simulink model "MJAUV_Maneuverability_model_V2"  (R2022b)
settings: Solver=ode4  StartTime=0.0  StopTime=50  FixedStep=0.0001  RelTol=1e-3  EnableMultiTasking=on
libraries: sharedutil x64, matrix_library x35
(part 4 of 5)

== system MJAUV_Maneuverability_model_V2/MJ-AUV Model & PropulsionSystem/Dynamics and Kinematics/Subsystem7/Rigid-body Coriolis and centripetal matrix1/Skew Symmetrical Operator  ==
  v : Inport
  Constant : Constant  Value=0
  Create 3x3 Matrix : sharedutil/Create 3x3 Matrix  aMode=aMode
  Demux : Demux  Outputs=3
      settings: DisplayOption=none
  Gain : Gain  Gain=-1  SaturateOnIntegerOverflow=on  OutDataTypeStr=Inherit: Same as input  ParamDataTypeStr=Inherit: Same as input
  Gain1 : Gain  Gain=-1  SaturateOnIntegerOverflow=on  OutDataTypeStr=Inherit: Same as input  ParamDataTypeStr=Inherit: Same as input
  Gain2 : Gain  Gain=-1  SaturateOnIntegerOverflow=on  OutDataTypeStr=Inherit: Same as input  ParamDataTypeStr=Inherit: Same as input
  S(V) : Outport  VectorParamsAs1DForOutWhenUnconnected=off
  wires:
  v/1 -> Demux/1
  Create 3x3 Matrix/1 -> S(V)/1
  Gain2/1 -> Create 3x3 Matrix/2  "-v(3)"
  Gain1/1 -> Create 3x3 Matrix/7  "-v(2)"
  Gain/1 -> Create 3x3 Matrix/6  "-v(1)"
  Demux/3 -> Create 3x3 Matrix/4, Gain2/1  "v(3)"
  Demux/2 -> Create 3x3 Matrix/3, Gain1/1  "v(2)"
  Demux/1 -> Create 3x3 Matrix/8, Gain/1  "v(1)"
  Constant/1 -> Create 3x3 Matrix/5, Create 3x3 Matrix/9, Create 3x3 Matrix/1

== system MJAUV_Maneuverability_model_V2/MJ-AUV Model & PropulsionSystem/Dynamics and Kinematics/Subsystem7/Rigid-body Coriolis and centripetal matrix1/Skew Symmetrical Operator ==
  v : Inport
  Constant : Constant  Value=0
  Create 3x3 Matrix : sharedutil/Create 3x3 Matrix  aMode=aMode
  Demux : Demux  Outputs=3
      settings: DisplayOption=none
  Gain : Gain  Gain=-1  SaturateOnIntegerOverflow=on  OutDataTypeStr=Inherit: Same as input  ParamDataTypeStr=Inherit: Same as input
  Gain1 : Gain  Gain=-1  SaturateOnIntegerOverflow=on  OutDataTypeStr=Inherit: Same as input  ParamDataTypeStr=Inherit: Same as input
  Gain2 : Gain  Gain=-1  SaturateOnIntegerOverflow=on  OutDataTypeStr=Inherit: Same as input  ParamDataTypeStr=Inherit: Same as input
  S(V) : Outport  VectorParamsAs1DForOutWhenUnconnected=off
  wires:
  v/1 -> Demux/1
  Create 3x3 Matrix/1 -> S(V)/1
  Gain2/1 -> Create 3x3 Matrix/2  "-v(3)"
  Gain1/1 -> Create 3x3 Matrix/7  "-v(2)"
  Gain/1 -> Create 3x3 Matrix/6  "-v(1)"
  Demux/3 -> Create 3x3 Matrix/4, Gain2/1  "v(3)"
  Demux/2 -> Create 3x3 Matrix/3, Gain1/1  "v(2)"
  Demux/1 -> Create 3x3 Matrix/8, Gain/1  "v(1)"
  Constant/1 -> Create 3x3 Matrix/5, Create 3x3 Matrix/9, Create 3x3 Matrix/1

== system MJAUV_Maneuverability_model_V2/MJ-AUV Model & PropulsionSystem/Dynamics and Kinematics/Subsystem7/Rigid-body Coriolis and centripetal matrix1/Skew Symmetrical Operator  ==
  v : Inport
  Constant : Constant  Value=0
  Create 3x3 Matrix : sharedutil/Create 3x3 Matrix  aMode=aMode
  Demux : Demux  Outputs=3
      settings: DisplayOption=none
  Gain : Gain  Gain=-1  SaturateOnIntegerOverflow=on  OutDataTypeStr=Inherit: Same as input  ParamDataTypeStr=Inherit: Same as input
  Gain1 : Gain  Gain=-1  SaturateOnIntegerOverflow=on  OutDataTypeStr=Inherit: Same as input  ParamDataTypeStr=Inherit: Same as input
  Gain2 : Gain  Gain=-1  SaturateOnIntegerOverflow=on  OutDataTypeStr=Inherit: Same as input  ParamDataTypeStr=Inherit: Same as input
  S(V) : Outport  VectorParamsAs1DForOutWhenUnconnected=off
  wires:
  Constant/1 -> Create 3x3 Matrix/1, Create 3x3 Matrix/9, Create 3x3 Matrix/5
  Demux/1 -> Gain/1, Create 3x3 Matrix/8  "v(1)"
  Demux/2 -> Gain1/1, Create 3x3 Matrix/3  "v(2)"
  Demux/3 -> Gain2/1, Create 3x3 Matrix/4  "v(3)"
  Gain/1 -> Create 3x3 Matrix/6  "-v(1)"
  Gain1/1 -> Create 3x3 Matrix/7  "-v(2)"
  Gain2/1 -> Create 3x3 Matrix/2  "-v(3)"
  Create 3x3 Matrix/1 -> S(V)/1
  v/1 -> Demux/1

== system MJAUV_Maneuverability_model_V2/MJ-AUV Model & PropulsionSystem/Dynamics and Kinematics/Subsystem7/Rigid-body Coriolis and centripetal matrix1/Skew Symmetrical Operator   ==
  v : Inport
  Constant : Constant  Value=0
  Create 3x3 Matrix : sharedutil/Create 3x3 Matrix  aMode=aMode
  Demux : Demux  Outputs=3
      settings: DisplayOption=none
  Gain : Gain  Gain=-1  SaturateOnIntegerOverflow=on  OutDataTypeStr=Inherit: Same as input  ParamDataTypeStr=Inherit: Same as input
  Gain1 : Gain  Gain=-1  SaturateOnIntegerOverflow=on  OutDataTypeStr=Inherit: Same as input  ParamDataTypeStr=Inherit: Same as input
  Gain2 : Gain  Gain=-1  SaturateOnIntegerOverflow=on  OutDataTypeStr=Inherit: Same as input  ParamDataTypeStr=Inherit: Same as input
  S(V) : Outport  VectorParamsAs1DForOutWhenUnconnected=off
  wires:
  v/1 -> Demux/1
  Create 3x3 Matrix/1 -> S(V)/1
  Gain2/1 -> Create 3x3 Matrix/2  "-v(3)"
  Gain1/1 -> Create 3x3 Matrix/7  "-v(2)"
  Gain/1 -> Create 3x3 Matrix/6  "-v(1)"
  Demux/3 -> Create 3x3 Matrix/4, Gain2/1  "v(3)"
  Demux/2 -> Create 3x3 Matrix/3, Gain1/1  "v(2)"
  Demux/1 -> Create 3x3 Matrix/8, Gain/1  "v(1)"
  Constant/1 -> Create 3x3 Matrix/5, Create 3x3 Matrix/9, Create 3x3 Matrix/1

== system MJAUV_Maneuverability_model_V2/MJ-AUV Model & PropulsionSystem/Dynamics and Kinematics/Subsystem7/Rigid-body Coriolis and centripetal matrix1/Subsystem ==
  rG_T : Inport
  Add : Sum
  Constant2 : Constant  Value=IT
  Gain5 : Gain  Gain=-mT
  Matrix Multiply4 : Product  Multiplication=Matrix(*)
  Skew Symmetrical Operator1 : Subsystem
  Ib_T : Outport
  wires:
  rG_T/1 -> Skew Symmetrical Operator1/1(v)  "rG_T"
  Constant2/1 -> Add/1
  Gain5/1 -> Add/2
  Matrix Multiply4/1 -> Gain5/1
  Skew Symmetrical Operator1/1(S(V)) -> Matrix Multiply4/1, Matrix Multiply4/2  "skewsymm(rG_T)"
  Add/1 -> Ib_T/1  "Ib_T"

== system MJAUV_Maneuverability_model_V2/MJ-AUV Model & PropulsionSystem/Dynamics and Kinematics/Subsystem7/Subsystem1/Quaternion normalisation ==
  eta_E : Inport
  Mux : Mux  Inputs=2
  Product : Product  Inputs=*/  SaturateOnIntegerOverflow=on  OutDataTypeStr=Inherit: Same as first input
  Reshape : Reshape  OutputDimensionality=Column vector (2-D)
  Selector : Selector  InputPortWidth=7  IndexOptions=Index vector (dialog)  Indices=[1 2 3]  OutputSizes=1
  Selector1 : Selector  InputPortWidth=7  IndexOptions=Index vector (dialog)  Indices=[4 5 6 7]  OutputSizes=1
  norm 1x4 vector : Subsystem
  eta_E (norm) : Outport  VectorParamsAs1DForOutWhenUnconnected=off
  wires:
  norm 1x4 vector/1(norm) -> Product/2
  Reshape/1 -> eta_E (norm)/1
  Mux/1 -> Reshape/1
  Product/1 -> Mux/2
  Selector/1 -> Mux/1
  Selector1/1 -> Product/1, norm 1x4 vector/1(Inport)
  eta_E/1 -> Selector/1, Selector1/1  "eta_E"

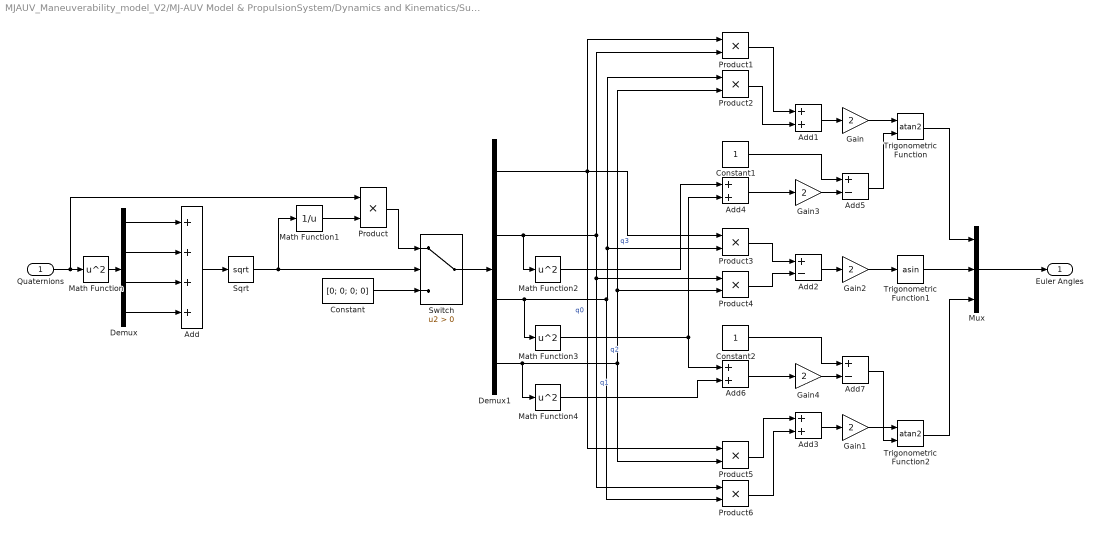
== system MJAUV_Maneuverability_model_V2/MJ-AUV Model & PropulsionSystem/Dynamics and Kinematics/Subsystem7/Subsystem1/Quaternions to Euler Angles ==
  Quaternions : Inport
  Add : Sum  Inputs=4
  Add{1,3..4,6} (4 alike) : Sum
  Add2 : Sum  Inputs=+-
  Add5 : Sum  Inputs=+-
  Add7 : Sum  Inputs=+-
  Constant : Constant  Value=[0; 0; 0; 0]
  Constant1 : Constant
  Constant2 : Constant
  Demux : Demux
  Demux1 : Demux
  Gain{,1..4} (5 alike) : Gain  Gain=2
  Math Function{,2..4} (4 alike) : Math  Operator=square  SignedPower=on
  Math Function1 : Math  Operator=reciprocal  SignedPower=on
  Mux : Mux  Inputs=3
  Product{,1..6} (7 alike) : Product
  Sqrt : Sqrt
  Switch : Switch  Criteria=u2 > Threshold  SaturateOnIntegerOverflow=off  InputSameDT=off
  Trigonometric Function : Trigonometry  Operator=atan2
  Trigonometric Function1 : Trigonometry  Operator=asin
  Trigonometric Function2 : Trigonometry  Operator=atan2
  Euler Angles : Outport  VectorParamsAs1DForOutWhenUnconnected=off
  wires:
  Quaternions/1 -> Product/1, Math Function/1
  Add/1 -> Sqrt/1
  Sqrt/1 -> Math Function1/1, Switch/2
  Constant/1 -> Switch/3
  Math Function1/1 -> Product/2
  Product/1 -> Switch/1
  Switch/1 -> Demux1/1
  Demux1/1 -> Product5/1, Product3/1, Product1/1  "q0"
  Demux1/2 -> Product6/1, Product4/1, Product1/2, Math Function2/1  "q1"
  Demux1/3 -> Product6/2, Product3/2, Product2/1, Math Function3/1  "q2"
  Demux1/4 -> Product5/2, Product4/2, Product2/2, Math Function4/1  "q3"
  Trigonometric Function1/1 -> Mux/2
  Mux/1 -> Euler Angles/1
  Trigonometric Function/1 -> Mux/1
  Trigonometric Function2/1 -> Mux/3
  Gain/1 -> Trigonometric Function/1
  Gain1/1 -> Trigonometric Function2/1
  Gain2/1 -> Trigonometric Function1/1
  Add1/1 -> Gain/1
  Add2/1 -> Gain2/1
  Add3/1 -> Gain1/1
  Product3/1 -> Add2/1
  Product4/1 -> Add2/2
  Product5/1 -> Add3/1
  Product6/1 -> Add3/2
  Product2/1 -> Add1/2
  Product1/1 -> Add1/1
  Add4/1 -> Gain3/1
  Gain3/1 -> Add5/2
  Constant1/1 -> Add5/1
  Add5/1 -> Trigonometric Function/2
  Add7/1 -> Trigonometric Function2/2
  Add6/1 -> Gain4/1
  Gain4/1 -> Add7/2
  Constant2/1 -> Add7/1
  Math Function2/1 -> Add4/1
  Math Function3/1 -> Add6/1, Add4/2
  Math Function4/1 -> Add6/2
  Demux/1 -> Add/1
  Demux/2 -> Add/2
  Demux/3 -> Add/3
  Demux/4 -> Add/4
  Math Function/1 -> Demux/1

== system MJAUV_Maneuverability_model_V2/MJ-AUV Model & PropulsionSystem/Dynamics and Kinematics/Subsystem7/Subsystem1/Subsystem ==
  "Euler Angles " : Inport
  Add : Sum
  Add1 : Sum  Inputs=-+
  Add2 : Sum
  Add3 : Sum  Inputs=+-
  Demux : Demux  Outputs=3
  Demux1 : Demux  Outputs=3
  Gain : Gain  Gain=0.5
  Mux : Mux
  Product{,1..7} (8 alike) : Product  Inputs=3
  Trigonometric Function : Trigonometry
  Trigonometric Function1 : Trigonometry  Operator=cos
  Quaternions : Outport  VectorParamsAs1DForOutWhenUnconnected=off
  wires:
  Add3/1 -> Mux/4
  Add2/1 -> Mux/3
  Add/1 -> Mux/1
  Add1/1 -> Mux/2
  Mux/1 -> Quaternions/1
  Product7/1 -> Add3/2
  Product6/1 -> Add3/1
  Product5/1 -> Add2/2
  Product4/1 -> Add2/1
  Product3/1 -> Add1/2
  Product2/1 -> Add1/1
  Product1/1 -> Add/2
  Product/1 -> Add/1
  Demux1/3 -> Product5/3, Product1/3, Product3/3, Product7/3  "cos(Y/2)"
  Demux1/1 -> Product5/1, Product2/1, Product1/1, Product6/1  "cos(R/2)"
  Demux1/2 -> Product6/2, Product1/2, Product3/2, Product4/2  "cos(P/2)"
  Trigonometric Function1/1 -> Demux1/1
  Demux/3 -> Product/3, Product2/3, Product4/3, Product6/3  "sin(Y/2)"
  Demux/2 -> Product/2, Product2/2, Product5/2, Product7/2  "sin(P/2)"
  Demux/1 -> Product/1, Product3/1, Product4/1, Product7/1  "sin(R/2)"
  Trigonometric Function/1 -> Demux/1
  Gain/1 -> Trigonometric Function/1, Trigonometric Function1/1
  "Euler Angles "/1 -> Gain/1

== system MJAUV_Maneuverability_model_V2/MJ-AUV Model & PropulsionSystem/Dynamics and Kinematics/Subsystem7/Subsystem1/Subsystem1 ==
  In2 : Inport
  Abs : Abs  SaturateOnIntegerOverflow=off
  Add : Sum  Inputs=-+
  Constant : Constant  Value=2*pi
  Switch : Switch  Criteria=u2 > Threshold  Threshold=pi  SaturateOnIntegerOverflow=off  InputSameDT=off
  Out1 : Outport
  wires:
  In2/1 -> Add/2, Switch/3, Abs/1
  Switch/1 -> Out1/1
  Add/1 -> Switch/1
  Abs/1 -> Switch/2
  Constant/1 -> Add/1

== system MJAUV_Maneuverability_model_V2/MJ-AUV Model & PropulsionSystem/Dynamics and Kinematics/Subsystem8/Added Mass Coriolis and centripetal matrix1/Skew Symmetrical Operator ==
  v : Inport
  Constant : Constant  Value=0
  Create 3x3 Matrix : sharedutil/Create 3x3 Matrix  aMode=aMode
  Demux : Demux  Outputs=3
      settings: DisplayOption=none
  Gain : Gain  Gain=-1  SaturateOnIntegerOverflow=on  OutDataTypeStr=Inherit: Same as input  ParamDataTypeStr=Inherit: Same as input
  Gain1 : Gain  Gain=-1  SaturateOnIntegerOverflow=on  OutDataTypeStr=Inherit: Same as input  ParamDataTypeStr=Inherit: Same as input
  Gain2 : Gain  Gain=-1  SaturateOnIntegerOverflow=on  OutDataTypeStr=Inherit: Same as input  ParamDataTypeStr=Inherit: Same as input
  S(V) : Outport  VectorParamsAs1DForOutWhenUnconnected=off
  wires:
  v/1 -> Demux/1
  Create 3x3 Matrix/1 -> S(V)/1
  Gain2/1 -> Create 3x3 Matrix/2  "-v(3)"
  Gain1/1 -> Create 3x3 Matrix/7  "-v(2)"
  Gain/1 -> Create 3x3 Matrix/6  "-v(1)"
  Demux/3 -> Create 3x3 Matrix/4, Gain2/1  "v(3)"
  Demux/2 -> Create 3x3 Matrix/3, Gain1/1  "v(2)"
  Demux/1 -> Create 3x3 Matrix/8, Gain/1  "v(1)"
  Constant/1 -> Create 3x3 Matrix/5, Create 3x3 Matrix/9, Create 3x3 Matrix/1

== system MJAUV_Maneuverability_model_V2/MJ-AUV Model & PropulsionSystem/Dynamics and Kinematics/Subsystem8/Added Mass Coriolis and centripetal matrix1/Skew Symmetrical Operator  ==
  v : Inport
  Constant : Constant  Value=0
  Create 3x3 Matrix : sharedutil/Create 3x3 Matrix  aMode=aMode
  Demux : Demux  Outputs=3
      settings: DisplayOption=none
  Gain : Gain  Gain=-1  SaturateOnIntegerOverflow=on  OutDataTypeStr=Inherit: Same as input  ParamDataTypeStr=Inherit: Same as input
  Gain1 : Gain  Gain=-1  SaturateOnIntegerOverflow=on  OutDataTypeStr=Inherit: Same as input  ParamDataTypeStr=Inherit: Same as input
  Gain2 : Gain  Gain=-1  SaturateOnIntegerOverflow=on  OutDataTypeStr=Inherit: Same as input  ParamDataTypeStr=Inherit: Same as input
  S(V) : Outport  VectorParamsAs1DForOutWhenUnconnected=off
  wires:
  Constant/1 -> Create 3x3 Matrix/1, Create 3x3 Matrix/9, Create 3x3 Matrix/5
  Demux/1 -> Gain/1, Create 3x3 Matrix/8  "v(1)"
  Demux/2 -> Gain1/1, Create 3x3 Matrix/3  "v(2)"
  Demux/3 -> Gain2/1, Create 3x3 Matrix/4  "v(3)"
  Gain/1 -> Create 3x3 Matrix/6  "-v(1)"
  Gain1/1 -> Create 3x3 Matrix/7  "-v(2)"
  Gain2/1 -> Create 3x3 Matrix/2  "-v(3)"
  Create 3x3 Matrix/1 -> S(V)/1
  v/1 -> Demux/1

== system MJAUV_Maneuverability_model_V2/MJ-AUV Model & PropulsionSystem/Dynamics and Kinematics/Subsystem8/Added Mass Coriolis and centripetal matrix1/Subsystem ==
  Create Diagonal Matrix1 : matrix_library/Create Diagonal Matrix
  K_pdot_F : Constant  Value=0
  M_qdot_F : Constant  Value=(pi*rho*R^2*LF^3)/12
  Mux : Mux  Inputs=6
  N_rdot_F : Constant  Value=(pi*rho*R^2*LF^3)/12
  Reshape1 : Reshape  OutputDimensionality=Column vector (2-D)  OutputDimensions=[6,6]
  X_udot_F : Constant  Value=0.1*mF
  Y_vdot_F : Constant  Value=pi*rho*R*R*LF
  Z_wdot_F : Constant  Value=pi*rho*R^2*LF
  MA_F : Outport
  wires:
  Create Diagonal Matrix1/1 -> MA_F/1
  K_pdot_F/1 -> Mux/4
  N_rdot_F/1 -> Mux/6
  M_qdot_F/1 -> Mux/5
  X_udot_F/1 -> Mux/1
  Y_vdot_F/1 -> Mux/2
  Reshape1/1 -> Create Diagonal Matrix1/1
  Mux/1 -> Reshape1/1
  Z_wdot_F/1 -> Mux/3

== system MJAUV_Maneuverability_model_V2/MJ-AUV Model & PropulsionSystem/Dynamics and Kinematics/Subsystem8/Restoring forces1/E1(e) ==
  e : Inport
  Gain : Gain  Gain=2  SaturateOnIntegerOverflow=on  OutDataTypeStr=Inherit: Same as input  ParamDataTypeStr=Inherit: Same as input
  "Gain " : Gain  Gain=2  SaturateOnIntegerOverflow=on  OutDataTypeStr=Inherit: Same as input  ParamDataTypeStr=Inherit: Same as input
  I (3x3) : Constant  Value=eye(3)
  Matrix Multiply : Product  Multiplication=Matrix(*)
  Product : Product  SaturateOnIntegerOverflow=on  OutDataTypeStr=Inherit: Same as first input
  Selector : Selector  InputPortWidth=4  IndexOptions=Index vector (dialog)  Indices=[1]  OutputSizes=1
  Selector1 : Selector  InputPortWidth=4  IndexOptions=Index vector (dialog)  Indices=[2 3 4]  OutputSizes=1
  Skew Symmetrical Operator : Subsystem
  Sum : Sum  Inputs=+++  SaturateOnIntegerOverflow=on
  E1 : Outport  VectorParamsAs1DForOutWhenUnconnected=off
  wires:
  Sum/1 -> E1/1
  Gain/1 -> Sum/3
  Product/1 -> Sum/2
  I (3x3)/1 -> Sum/1
  "Gain "/1 -> Product/1
  Matrix Multiply/1 -> Gain/1
  Skew Symmetrical Operator/1(S(V)) -> Product/2, Matrix Multiply/2, Matrix Multiply/1
  Selector1/1 -> Skew Symmetrical Operator/1(v)  "eps"
  Selector/1 -> "Gain "/1  "eta"
  e/1 -> Selector1/1, Selector/1

== system MJAUV_Maneuverability_model_V2/MJ-AUV Model & PropulsionSystem/Dynamics and Kinematics/Subsystem8/Rigid-body Coriolis and centripetal matrix1/Ib_F ==
  rG_F : Inport
  Add : Sum
  Constant2 : Constant  Value=IF
  Gain5 : Gain  Gain=-mF
  Matrix Multiply4 : Product  Multiplication=Matrix(*)
  Skew Symmetrical Operator1 : Subsystem
  Ib_F : Outport
  wires:
  rG_F/1 -> Skew Symmetrical Operator1/1(v)  "rG_F"
  Constant2/1 -> Add/1
  Gain5/1 -> Add/2
  Matrix Multiply4/1 -> Gain5/1
  Skew Symmetrical Operator1/1(S(V)) -> Matrix Multiply4/1, Matrix Multiply4/2  "skewsymm(rG_F)"
  Add/1 -> Ib_F/1  "Ib_F"

== system MJAUV_Maneuverability_model_V2/MJ-AUV Model & PropulsionSystem/Dynamics and Kinematics/Subsystem8/Rigid-body Coriolis and centripetal matrix1/Skew Symmetrical Operator  ==
  v : Inport
  Constant : Constant  Value=0
  Create 3x3 Matrix : sharedutil/Create 3x3 Matrix  aMode=aMode
  Demux : Demux  Outputs=3
      settings: DisplayOption=none
  Gain : Gain  Gain=-1  SaturateOnIntegerOverflow=on  OutDataTypeStr=Inherit: Same as input  ParamDataTypeStr=Inherit: Same as input
  Gain1 : Gain  Gain=-1  SaturateOnIntegerOverflow=on  OutDataTypeStr=Inherit: Same as input  ParamDataTypeStr=Inherit: Same as input
  Gain2 : Gain  Gain=-1  SaturateOnIntegerOverflow=on  OutDataTypeStr=Inherit: Same as input  ParamDataTypeStr=Inherit: Same as input
  S(V) : Outport  VectorParamsAs1DForOutWhenUnconnected=off
  wires:
  Constant/1 -> Create 3x3 Matrix/1, Create 3x3 Matrix/9, Create 3x3 Matrix/5
  Demux/1 -> Gain/1, Create 3x3 Matrix/8  "v(1)"
  Demux/2 -> Gain1/1, Create 3x3 Matrix/3  "v(2)"
  Demux/3 -> Gain2/1, Create 3x3 Matrix/4  "v(3)"
  Gain/1 -> Create 3x3 Matrix/6  "-v(1)"
  Gain1/1 -> Create 3x3 Matrix/7  "-v(2)"
  Gain2/1 -> Create 3x3 Matrix/2  "-v(3)"
  Create 3x3 Matrix/1 -> S(V)/1
  v/1 -> Demux/1

== system MJAUV_Maneuverability_model_V2/MJ-AUV Model & PropulsionSystem/Dynamics and Kinematics/Subsystem8/Rigid-body Coriolis and centripetal matrix1/Skew Symmetrical Operator ==
  v : Inport
  Constant : Constant  Value=0
  Create 3x3 Matrix : sharedutil/Create 3x3 Matrix  aMode=aMode
  Demux : Demux  Outputs=3
      settings: DisplayOption=none
  Gain : Gain  Gain=-1  SaturateOnIntegerOverflow=on  OutDataTypeStr=Inherit: Same as input  ParamDataTypeStr=Inherit: Same as input
  Gain1 : Gain  Gain=-1  SaturateOnIntegerOverflow=on  OutDataTypeStr=Inherit: Same as input  ParamDataTypeStr=Inherit: Same as input
  Gain2 : Gain  Gain=-1  SaturateOnIntegerOverflow=on  OutDataTypeStr=Inherit: Same as input  ParamDataTypeStr=Inherit: Same as input
  S(V) : Outport  VectorParamsAs1DForOutWhenUnconnected=off
  wires:
  Constant/1 -> Create 3x3 Matrix/1, Create 3x3 Matrix/9, Create 3x3 Matrix/5
  Demux/1 -> Gain/1, Create 3x3 Matrix/8  "v(1)"
  Demux/2 -> Gain1/1, Create 3x3 Matrix/3  "v(2)"
  Demux/3 -> Gain2/1, Create 3x3 Matrix/4  "v(3)"
  Gain/1 -> Create 3x3 Matrix/6  "-v(1)"
  Gain1/1 -> Create 3x3 Matrix/7  "-v(2)"
  Gain2/1 -> Create 3x3 Matrix/2  "-v(3)"
  Create 3x3 Matrix/1 -> S(V)/1
  v/1 -> Demux/1

== system MJAUV_Maneuverability_model_V2/MJ-AUV Model & PropulsionSystem/Dynamics and Kinematics/Subsystem8/Rigid-body Coriolis and centripetal matrix1/Skew Symmetrical Operator  ==
  v : Inport
  Constant : Constant  Value=0
  Create 3x3 Matrix : sharedutil/Create 3x3 Matrix  aMode=aMode
  Demux : Demux  Outputs=3
      settings: DisplayOption=none
  Gain : Gain  Gain=-1  SaturateOnIntegerOverflow=on  OutDataTypeStr=Inherit: Same as input  ParamDataTypeStr=Inherit: Same as input
  Gain1 : Gain  Gain=-1  SaturateOnIntegerOverflow=on  OutDataTypeStr=Inherit: Same as input  ParamDataTypeStr=Inherit: Same as input
  Gain2 : Gain  Gain=-1  SaturateOnIntegerOverflow=on  OutDataTypeStr=Inherit: Same as input  ParamDataTypeStr=Inherit: Same as input
  S(V) : Outport  VectorParamsAs1DForOutWhenUnconnected=off
  wires:
  v/1 -> Demux/1
  Create 3x3 Matrix/1 -> S(V)/1
  Gain2/1 -> Create 3x3 Matrix/2  "-v(3)"
  Gain1/1 -> Create 3x3 Matrix/7  "-v(2)"
  Gain/1 -> Create 3x3 Matrix/6  "-v(1)"
  Demux/3 -> Create 3x3 Matrix/4, Gain2/1  "v(3)"
  Demux/2 -> Create 3x3 Matrix/3, Gain1/1  "v(2)"
  Demux/1 -> Create 3x3 Matrix/8, Gain/1  "v(1)"
  Constant/1 -> Create 3x3 Matrix/5, Create 3x3 Matrix/9, Create 3x3 Matrix/1

== system MJAUV_Maneuverability_model_V2/MJ-AUV Model & PropulsionSystem/Dynamics and Kinematics/Subsystem8/Rigid-body Coriolis and centripetal matrix1/Skew Symmetrical Operator   ==
  v : Inport
  Constant : Constant  Value=0
  Create 3x3 Matrix : sharedutil/Create 3x3 Matrix  aMode=aMode
  Demux : Demux  Outputs=3
      settings: DisplayOption=none
  Gain : Gain  Gain=-1  SaturateOnIntegerOverflow=on  OutDataTypeStr=Inherit: Same as input  ParamDataTypeStr=Inherit: Same as input
  Gain1 : Gain  Gain=-1  SaturateOnIntegerOverflow=on  OutDataTypeStr=Inherit: Same as input  ParamDataTypeStr=Inherit: Same as input
  Gain2 : Gain  Gain=-1  SaturateOnIntegerOverflow=on  OutDataTypeStr=Inherit: Same as input  ParamDataTypeStr=Inherit: Same as input
  S(V) : Outport  VectorParamsAs1DForOutWhenUnconnected=off
  wires:
  Constant/1 -> Create 3x3 Matrix/1, Create 3x3 Matrix/9, Create 3x3 Matrix/5
  Demux/1 -> Gain/1, Create 3x3 Matrix/8  "v(1)"
  Demux/2 -> Gain1/1, Create 3x3 Matrix/3  "v(2)"
  Demux/3 -> Gain2/1, Create 3x3 Matrix/4  "v(3)"
  Gain/1 -> Create 3x3 Matrix/6  "-v(1)"
  Gain1/1 -> Create 3x3 Matrix/7  "-v(2)"
  Gain2/1 -> Create 3x3 Matrix/2  "-v(3)"
  Create 3x3 Matrix/1 -> S(V)/1
  v/1 -> Demux/1

== system MJAUV_Maneuverability_model_V2/MJ-AUV Model & PropulsionSystem/Dynamics and Kinematics/Subsystem8/Subsystem1/Quaternion normalisation ==
  eta_E : Inport
  Mux : Mux  Inputs=2
  Product : Product  Inputs=*/  SaturateOnIntegerOverflow=on  OutDataTypeStr=Inherit: Same as first input
  Reshape : Reshape  OutputDimensionality=Column vector (2-D)
  Selector : Selector  InputPortWidth=7  IndexOptions=Index vector (dialog)  Indices=[1 2 3]  OutputSizes=1
  Selector1 : Selector  InputPortWidth=7  IndexOptions=Index vector (dialog)  Indices=[4 5 6 7]  OutputSizes=1
  norm 1x4 vector : Subsystem
  eta_E (norm) : Outport  VectorParamsAs1DForOutWhenUnconnected=off
  wires:
  norm 1x4 vector/1(norm) -> Product/2
  Reshape/1 -> eta_E (norm)/1
  Mux/1 -> Reshape/1
  Product/1 -> Mux/2
  Selector/1 -> Mux/1
  Selector1/1 -> Product/1, norm 1x4 vector/1(Inport)
  eta_E/1 -> Selector/1, Selector1/1  "eta_E"

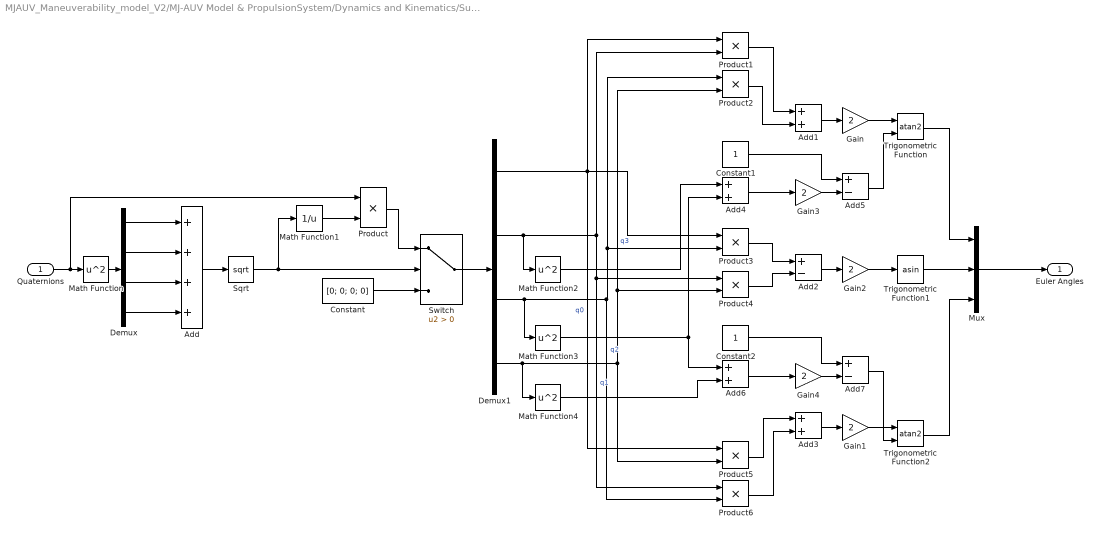
== system MJAUV_Maneuverability_model_V2/MJ-AUV Model & PropulsionSystem/Dynamics and Kinematics/Subsystem8/Subsystem1/Quaternions to Euler Angles ==
  Quaternions : Inport
  Add : Sum  Inputs=4
  Add{1,3..4,6} (4 alike) : Sum
  Add2 : Sum  Inputs=+-
  Add5 : Sum  Inputs=+-
  Add7 : Sum  Inputs=+-
  Constant : Constant  Value=[0; 0; 0; 0]
  Constant1 : Constant
  Constant2 : Constant
  Demux : Demux
  Demux1 : Demux
  Gain{,1..4} (5 alike) : Gain  Gain=2
  Math Function{,2..4} (4 alike) : Math  Operator=square  SignedPower=on
  Math Function1 : Math  Operator=reciprocal  SignedPower=on
  Mux : Mux  Inputs=3
  Product{,1..6} (7 alike) : Product
  Sqrt : Sqrt
  Switch : Switch  Criteria=u2 > Threshold  SaturateOnIntegerOverflow=off  InputSameDT=off
  Trigonometric Function : Trigonometry  Operator=atan2
  Trigonometric Function1 : Trigonometry  Operator=asin
  Trigonometric Function2 : Trigonometry  Operator=atan2
  Euler Angles : Outport  VectorParamsAs1DForOutWhenUnconnected=off
  wires:
  Quaternions/1 -> Product/1, Math Function/1
  Add/1 -> Sqrt/1
  Sqrt/1 -> Math Function1/1, Switch/2
  Constant/1 -> Switch/3
  Math Function1/1 -> Product/2
  Product/1 -> Switch/1
  Switch/1 -> Demux1/1
  Demux1/1 -> Product5/1, Product3/1, Product1/1  "q0"
  Demux1/2 -> Product6/1, Product4/1, Product1/2, Math Function2/1  "q1"
  Demux1/3 -> Product6/2, Product3/2, Product2/1, Math Function3/1  "q2"
  Demux1/4 -> Product5/2, Product4/2, Product2/2, Math Function4/1  "q3"
  Trigonometric Function1/1 -> Mux/2
  Mux/1 -> Euler Angles/1
  Trigonometric Function/1 -> Mux/1
  Trigonometric Function2/1 -> Mux/3
  Gain/1 -> Trigonometric Function/1
  Gain1/1 -> Trigonometric Function2/1
  Gain2/1 -> Trigonometric Function1/1
  Add1/1 -> Gain/1
  Add2/1 -> Gain2/1
  Add3/1 -> Gain1/1
  Product3/1 -> Add2/1
  Product4/1 -> Add2/2
  Product5/1 -> Add3/1
  Product6/1 -> Add3/2
  Product2/1 -> Add1/2
  Product1/1 -> Add1/1
  Add4/1 -> Gain3/1
  Gain3/1 -> Add5/2
  Constant1/1 -> Add5/1
  Add5/1 -> Trigonometric Function/2
  Add7/1 -> Trigonometric Function2/2
  Add6/1 -> Gain4/1
  Gain4/1 -> Add7/2
  Constant2/1 -> Add7/1
  Math Function2/1 -> Add4/1
  Math Function3/1 -> Add6/1, Add4/2
  Math Function4/1 -> Add6/2
  Demux/1 -> Add/1
  Demux/2 -> Add/2
  Demux/3 -> Add/3
  Demux/4 -> Add/4
  Math Function/1 -> Demux/1

== system MJAUV_Maneuverability_model_V2/MJ-AUV Model & PropulsionSystem/Dynamics and Kinematics/Subsystem8/Subsystem1/Subsystem ==
  "Euler Angles " : Inport
  Add : Sum
  Add1 : Sum  Inputs=-+
  Add2 : Sum
  Add3 : Sum  Inputs=+-
  Demux : Demux  Outputs=3
  Demux1 : Demux  Outputs=3
  Gain : Gain  Gain=0.5
  Mux : Mux
  Product{,1..7} (8 alike) : Product  Inputs=3
  Trigonometric Function : Trigonometry
  Trigonometric Function1 : Trigonometry  Operator=cos
  Quaternions : Outport  VectorParamsAs1DForOutWhenUnconnected=off
  wires:
  Add3/1 -> Mux/4
  Add2/1 -> Mux/3
  Add/1 -> Mux/1
  Add1/1 -> Mux/2
  Mux/1 -> Quaternions/1
  Product7/1 -> Add3/2
  Product6/1 -> Add3/1
  Product5/1 -> Add2/2
  Product4/1 -> Add2/1
  Product3/1 -> Add1/2
  Product2/1 -> Add1/1
  Product1/1 -> Add/2
  Product/1 -> Add/1
  Demux1/3 -> Product5/3, Product1/3, Product3/3, Product7/3  "cos(Y/2)"
  Demux1/1 -> Product5/1, Product2/1, Product1/1, Product6/1  "cos(R/2)"
  Demux1/2 -> Product6/2, Product1/2, Product3/2, Product4/2  "cos(P/2)"
  Trigonometric Function1/1 -> Demux1/1
  Demux/3 -> Product/3, Product2/3, Product4/3, Product6/3  "sin(Y/2)"
  Demux/2 -> Product/2, Product2/2, Product5/2, Product7/2  "sin(P/2)"
  Demux/1 -> Product/1, Product3/1, Product4/1, Product7/1  "sin(R/2)"
  Trigonometric Function/1 -> Demux/1
  Gain/1 -> Trigonometric Function/1, Trigonometric Function1/1
  "Euler Angles "/1 -> Gain/1

== system MJAUV_Maneuverability_model_V2/MJ-AUV Model & PropulsionSystem/Dynamics and Kinematics/Subsystem8/Subsystem1/Subsystem1 ==
  In2 : Inport
  Abs : Abs  SaturateOnIntegerOverflow=off
  Add : Sum  Inputs=-+
  Constant : Constant  Value=2*pi
  Switch : Switch  Criteria=u2 > Threshold  Threshold=pi  SaturateOnIntegerOverflow=off  InputSameDT=off
  Out1 : Outport
  wires:
  In2/1 -> Add/2, Switch/3, Abs/1
  Switch/1 -> Out1/1
  Add/1 -> Switch/1
  Abs/1 -> Switch/2
  Constant/1 -> Add/1

== system MJAUV_Maneuverability_model_V2/MJ-AUV Model & PropulsionSystem/Dynamics and Kinematics/Subsystem9/M_B/Subsystem ==
  Create Diagonal Matrix1 : matrix_library/Create Diagonal Matrix
  K_pdot_B : Constant  Value=0
  M_qdot_B : Constant  Value=(pi*rho*R^2*LB^3)/12
  Mux : Mux  Inputs=6
  N_rdot_B : Constant  Value=(pi*rho*R^2*LB^3)/12
  Reshape1 : Reshape  OutputDimensionality=Column vector (2-D)  OutputDimensions=[6,6]
  X_udot_B : Constant  Value=0.1*mB
  Y_vdot_B : Constant  Value=pi*rho*R*R*LB
  Z_wdot_B : Constant  Value=pi*rho*R^2*LB
  MA_B : Outport
  wires:
  Create Diagonal Matrix1/1 -> MA_B/1
  K_pdot_B/1 -> Mux/4
  N_rdot_B/1 -> Mux/6
  M_qdot_B/1 -> Mux/5
  X_udot_B/1 -> Mux/1
  Y_vdot_B/1 -> Mux/2
  Reshape1/1 -> Create Diagonal Matrix1/1
  Mux/1 -> Reshape1/1
  Z_wdot_B/1 -> Mux/3

== system MJAUV_Maneuverability_model_V2/MJ-AUV Model & PropulsionSystem/Dynamics and Kinematics/Subsystem9/M_B/Subsystem1 ==
  rG_B : Inport
  Add : Sum
  Constant2 : Constant  Value=IB
  Gain : Gain  Gain=-mB
  Gain1 : Gain  Gain=-1
  Gain2 : Gain  Gain=-mB
  Gain3 : Gain  Gain=mB
  Matrix Concatenation : Concatenate  Mode=Multidimensional array
  Matrix Concatenation1 : Concatenate  Mode=Multidimensional array
  Matrix Concatenation2 : Concatenate  Mode=Multidimensional array  ConcatenateDimension=2
  Matrix Multiply3 : Product  Multiplication=Matrix(*)
  Skew Symmetrical Operator1 : Subsystem
  eye(3,3) : Constant  Value=eye(3,3)
  MRB_B : Outport  VectorParamsAs1DForOutWhenUnconnected=off
  wires:
  Matrix Concatenation2/1 -> MRB_B/1
  Gain2/1 -> Add/2
  Skew Symmetrical Operator1/1(S(V)) -> Gain/1, Matrix Multiply3/2, Matrix Multiply3/1  "skewsymm(rG_B)"
  Gain3/1 -> Matrix Concatenation/1  "MRB_B(1,1)"
  eye(3,3)/1 -> Gain3/1  "eye(3,3)"
  Gain1/1 -> Matrix Concatenation1/1  "MRB_B(2,1)"
  Add/1 -> Matrix Concatenation1/2  "MRB_B(2,2)"
  Matrix Concatenation/1 -> Matrix Concatenation2/1
  Matrix Concatenation1/1 -> Matrix Concatenation2/2
  Gain/1 -> Matrix Concatenation/2, Gain1/1  "MRB_B(1,2)"
  Matrix Multiply3/1 -> Gain2/1
  Constant2/1 -> Add/1
  rG_B/1 -> Skew Symmetrical Operator1/1(v)

== system MJAUV_Maneuverability_model_V2/MJ-AUV Model & PropulsionSystem/Dynamics and Kinematics/Subsystem9/M_F/Subsystem ==
  Create Diagonal Matrix1 : matrix_library/Create Diagonal Matrix
  K_pdot_F : Constant  Value=0
  M_qdot_F : Constant  Value=(pi*rho*R^2*LF^3)/12
  Mux : Mux  Inputs=6
  N_rdot_F : Constant  Value=(pi*rho*R^2*LF^3)/12
  Reshape1 : Reshape  OutputDimensionality=Column vector (2-D)  OutputDimensions=[6,6]
  X_udot_F : Constant  Value=0.1*mF
  Y_vdot_F : Constant  Value=pi*rho*R*R*LF
  Z_wdot_F : Constant  Value=pi*rho*R^2*LF
  MA_F : Outport
  wires:
  Create Diagonal Matrix1/1 -> MA_F/1
  K_pdot_F/1 -> Mux/4
  N_rdot_F/1 -> Mux/6
  M_qdot_F/1 -> Mux/5
  X_udot_F/1 -> Mux/1
  Y_vdot_F/1 -> Mux/2
  Reshape1/1 -> Create Diagonal Matrix1/1
  Mux/1 -> Reshape1/1
  Z_wdot_F/1 -> Mux/3

== system MJAUV_Maneuverability_model_V2/MJ-AUV Model & PropulsionSystem/Dynamics and Kinematics/Subsystem9/M_F/Subsystem1 ==
  rG_F : Inport
  Add : Sum
  Constant2 : Constant  Value=IF
  Gain : Gain  Gain=-mF
  Gain1 : Gain  Gain=-1
  Gain2 : Gain  Gain=-mF
  Gain3 : Gain  Gain=mF
  Matrix Concatenation : Concatenate  Mode=Multidimensional array
  Matrix Concatenation1 : Concatenate  Mode=Multidimensional array
  Matrix Concatenation2 : Concatenate  Mode=Multidimensional array  ConcatenateDimension=2
  Matrix Multiply3 : Product  Multiplication=Matrix(*)
  Skew Symmetrical Operator1 : Subsystem
  eye(3,3) : Constant  Value=eye(3,3)
  MRB_F : Outport  VectorParamsAs1DForOutWhenUnconnected=off
  wires:
  Matrix Concatenation2/1 -> MRB_F/1
  Gain2/1 -> Add/2
  Skew Symmetrical Operator1/1(S(V)) -> Gain/1, Matrix Multiply3/2, Matrix Multiply3/1  "skewsymm(rG_F)"
  Gain3/1 -> Matrix Concatenation/1  "MRB_F(1,1)"
  eye(3,3)/1 -> Gain3/1  "eye(3,3)"
  Gain1/1 -> Matrix Concatenation1/1  "MRB_F(2,1)"
  Add/1 -> Matrix Concatenation1/2  "MRB_F(2,2)"
  Matrix Concatenation/1 -> Matrix Concatenation2/1
  Matrix Concatenation1/1 -> Matrix Concatenation2/2
  Gain/1 -> Gain1/1, Matrix Concatenation/2  "MRB_F(1,2)"
  Matrix Multiply3/1 -> Gain2/1
  Constant2/1 -> Add/1
  rG_F/1 -> Skew Symmetrical Operator1/1(v)

== system MJAUV_Maneuverability_model_V2/MJ-AUV Model & PropulsionSystem/Dynamics and Kinematics/Subsystem9/M_S/Subsystem ==
  Create Diagonal Matrix1 : matrix_library/Create Diagonal Matrix
  K_pdot_S : Constant  Value=0
  M_qdot_S : Constant  Value=(pi*rho*R^2*LS^3)/12
  Mux : Mux  Inputs=6
  N_rdot_S : Constant  Value=(pi*rho*R^2*LS^3)/12
  Reshape1 : Reshape  OutputDimensionality=Column vector (2-D)  OutputDimensions=[6,6]
  X_udot_S : Constant  Value=0.1*mS
  Y_vdot_S : Constant  Value=pi*rho*R*R*LS
  Z_wdot_S : Constant  Value=pi*rho*R^2*LS
  MA_S : Outport
  wires:
  Z_wdot_S/1 -> Mux/3
  Mux/1 -> Reshape1/1
  Reshape1/1 -> Create Diagonal Matrix1/1
  Y_vdot_S/1 -> Mux/2
  X_udot_S/1 -> Mux/1
  M_qdot_S/1 -> Mux/5
  N_rdot_S/1 -> Mux/6
  K_pdot_S/1 -> Mux/4
  Create Diagonal Matrix1/1 -> MA_S/1

== system MJAUV_Maneuverability_model_V2/MJ-AUV Model & PropulsionSystem/Dynamics and Kinematics/Subsystem9/M_S/Subsystem1 ==
  rG_S : Inport
  Add : Sum
  Constant2 : Constant  Value=IS
  Gain : Gain  Gain=-mS
  Gain1 : Gain  Gain=-1
  Gain2 : Gain  Gain=-mS
  Gain3 : Gain  Gain=mS
  Matrix Concatenation : Concatenate  Mode=Multidimensional array
  Matrix Concatenation1 : Concatenate  Mode=Multidimensional array
  Matrix Concatenation2 : Concatenate  Mode=Multidimensional array  ConcatenateDimension=2
  Matrix Multiply3 : Product  Multiplication=Matrix(*)
  Skew Symmetrical Operator1 : Subsystem
  eye(3,3) : Constant  Value=eye(3,3)
  MRB_S : Outport  VectorParamsAs1DForOutWhenUnconnected=off
  wires:
  rG_S/1 -> Skew Symmetrical Operator1/1(v)
  Constant2/1 -> Add/1
  Matrix Multiply3/1 -> Gain2/1
  Gain/1 -> Matrix Concatenation/2, Gain1/1  "MRB_S(1,2)"
  Matrix Concatenation1/1 -> Matrix Concatenation2/2
  Matrix Concatenation/1 -> Matrix Concatenation2/1
  Add/1 -> Matrix Concatenation1/2  "MRB_S(2,2)"
  Gain1/1 -> Matrix Concatenation1/1  "MRB_S(2,1)"
  eye(3,3)/1 -> Gain3/1  "eye(3,3)"
  Gain3/1 -> Matrix Concatenation/1  "MRB_S(1,1)"
  Skew Symmetrical Operator1/1(S(V)) -> Matrix Multiply3/1, Matrix Multiply3/2, Gain/1  "skewsymm(rG_S)"
  Gain2/1 -> Add/2
  Matrix Concatenation2/1 -> MRB_S/1

== system MJAUV_Maneuverability_model_V2/MJ-AUV Model & PropulsionSystem/Dynamics and Kinematics/Subsystem9/M_T/Subsystem ==
  Create Diagonal Matrix1 : matrix_library/Create Diagonal Matrix
  K_pdot_T : Constant  Value=0
  M_qdot_T : Constant  Value=(pi*rho*R^2*LT^3)/12
  Mux : Mux  Inputs=6
  N_rdot_T : Constant  Value=(pi*rho*R^2*LT^3)/12
  Reshape1 : Reshape  OutputDimensionality=Column vector (2-D)  OutputDimensions=[6,6]
  X_udot_T : Constant  Value=0.1*mT
  Y_vdot_T : Constant  Value=pi*rho*R*R*LT
  Z_wdot_T : Constant  Value=pi*rho*R^2*LT
  MA_T : Outport
  wires:
  Z_wdot_T/1 -> Mux/3
  Mux/1 -> Reshape1/1
  Reshape1/1 -> Create Diagonal Matrix1/1
  Y_vdot_T/1 -> Mux/2
  X_udot_T/1 -> Mux/1
  M_qdot_T/1 -> Mux/5
  N_rdot_T/1 -> Mux/6
  K_pdot_T/1 -> Mux/4
  Create Diagonal Matrix1/1 -> MA_T/1

== system MJAUV_Maneuverability_model_V2/MJ-AUV Model & PropulsionSystem/Dynamics and Kinematics/Subsystem9/M_T/Subsystem1 ==
  rG_T : Inport
  Add : Sum
  Constant2 : Constant  Value=IT
  Gain : Gain  Gain=-mT
  Gain1 : Gain  Gain=-1
  Gain2 : Gain  Gain=-mT
  Gain3 : Gain  Gain=mT
  Matrix Concatenation : Concatenate  Mode=Multidimensional array
  Matrix Concatenation1 : Concatenate  Mode=Multidimensional array
  Matrix Concatenation2 : Concatenate  Mode=Multidimensional array  ConcatenateDimension=2
  Matrix Multiply3 : Product  Multiplication=Matrix(*)
  Skew Symmetrical Operator1 : Subsystem
  eye(3,3) : Constant  Value=eye(3,3)
  MRB_T : Outport  VectorParamsAs1DForOutWhenUnconnected=off
  wires:
  rG_T/1 -> Skew Symmetrical Operator1/1(v)
  Constant2/1 -> Add/1
  Matrix Multiply3/1 -> Gain2/1
  Gain/1 -> Matrix Concatenation/2, Gain1/1  "MRB_T(1,2)"
  Matrix Concatenation1/1 -> Matrix Concatenation2/2
  Matrix Concatenation/1 -> Matrix Concatenation2/1
  Add/1 -> Matrix Concatenation1/2  "MRB_T(2,2)"
  Gain1/1 -> Matrix Concatenation1/1  "MRB_T(2,1)"
  eye(3,3)/1 -> Gain3/1  "eye(3,3)"
  Gain3/1 -> Matrix Concatenation/1  "MRB_T(1,1)"
  Skew Symmetrical Operator1/1(S(V)) -> Matrix Multiply3/1, Matrix Multiply3/2, Gain/1  "skewsymm(rG_T)"
  Gain2/1 -> Add/2
  Matrix Concatenation2/1 -> MRB_T/1

== system MJAUV_Maneuverability_model_V2/MJ-AUV Model & PropulsionSystem/Dynamics and Kinematics/Subsystem9/Subsystem5/K ==
  R_FT : Inport
  Constant1 : Constant  Value=r_T
  Gain : Gain  Gain=-1
  Matrix Concatenation : Concatenate  Mode=Multidimensional array
  Matrix Concatenation1 : Concatenate  Mode=Multidimensional array
  Matrix Concatenation2 : Concatenate  Mode=Multidimensional array  ConcatenateDimension=2
  Matrix Multiply3 : Product  Multiplication=Matrix(*)
  "Skew Symmetrical Operator " : Subsystem
  Zero matrix (3 x 3) : Constant  Value=zeros(3,3)
  K_FT : Outport
  wires:
  Matrix Concatenation2/1 -> K_FT/1
  Zero matrix (3 x 3)/1 -> Matrix Concatenation1/1  "R(2,1)"
  Matrix Multiply3/1 -> Gain/1
  Matrix Concatenation1/1 -> Matrix Concatenation2/2
  Matrix Concatenation/1 -> Matrix Concatenation2/1
  R_FT/1 -> Matrix Multiply3/1, Matrix Concatenation/1, Matrix Concatenation1/2
  Gain/1 -> Matrix Concatenation/2  "R(1,2)"
  "Skew Symmetrical Operator "/1(S(V)) -> Matrix Multiply3/2
  Constant1/1 -> "Skew Symmetrical Operator "/1(v)

== system MJAUV_Maneuverability_model_V2/MJ-AUV Model & PropulsionSystem/Dynamics and Kinematics/Subsystem9/Subsystem5/K_B ==
  R_SB : Inport
  Constant1 : Constant  Value=r_B
  Gain : Gain  Gain=-1
  Matrix Concatenation : Concatenate  Mode=Multidimensional array
  Matrix Concatenation1 : Concatenate  Mode=Multidimensional array
  Matrix Concatenation2 : Concatenate  Mode=Multidimensional array  ConcatenateDimension=2
  Matrix Multiply3 : Product  Multiplication=Matrix(*)
  "Skew Symmetrical Operator " : Subsystem
  Zero matrix (3 x 3) : Constant  Value=zeros(3,3)
  K_SB : Outport
  wires:
  Constant1/1 -> "Skew Symmetrical Operator "/1(v)
  "Skew Symmetrical Operator "/1(S(V)) -> Matrix Multiply3/2
  Gain/1 -> Matrix Concatenation1/1  "R(1,2)"
  R_SB/1 -> Matrix Concatenation1/2, Matrix Concatenation/1, Matrix Multiply3/1
  Matrix Concatenation/1 -> Matrix Concatenation2/1
  Matrix Concatenation1/1 -> Matrix Concatenation2/2
  Matrix Multiply3/1 -> Gain/1
  Zero matrix (3 x 3)/1 -> Matrix Concatenation/2  "R(2,1)"
  Matrix Concatenation2/1 -> K_SB/1

== system MJAUV_Maneuverability_model_V2/MJ-AUV Model & PropulsionSystem/Dynamics and Kinematics/Subsystem9/Subsystem5/K_T ==
  R_TS : Inport
  Constant1 : Constant  Value=r_S
  Gain : Gain  Gain=-1
  Matrix Concatenation : Concatenate  Mode=Multidimensional array
  Matrix Concatenation1 : Concatenate  Mode=Multidimensional array
  Matrix Concatenation2 : Concatenate  Mode=Multidimensional array  ConcatenateDimension=2
  Matrix Multiply3 : Product  Multiplication=Matrix(*)
  "Skew Symmetrical Operator " : Subsystem
  Zero matrix (3 x 3) : Constant  Value=zeros(3,3)
  K_TS : Outport
  wires:
  Constant1/1 -> "Skew Symmetrical Operator "/1(v)
  "Skew Symmetrical Operator "/1(S(V)) -> Matrix Multiply3/2
  Gain/1 -> Matrix Concatenation1/1  "R(1,2)"
  R_TS/1 -> Matrix Concatenation1/2, Matrix Concatenation/1, Matrix Multiply3/1
  Matrix Concatenation/1 -> Matrix Concatenation2/1
  Matrix Concatenation1/1 -> Matrix Concatenation2/2
  Matrix Multiply3/1 -> Gain/1
  Zero matrix (3 x 3)/1 -> Matrix Concatenation/2  "R(2,1)"
  Matrix Concatenation2/1 -> K_TS/1

== system MJAUV_Maneuverability_model_V2/MJ-AUV Model & PropulsionSystem/Dynamics and Kinematics/Subsystem9/Subsystem5/{B}->{S} Transformation ==
  v : Inport
  Constant : Constant  Value=0
  Constant1 : Constant
  Create 3x3 Matrix : sharedutil/Create 3x3 Matrix  aMode=aMode
  Gain : Gain  Gain=-1  SaturateOnIntegerOverflow=on  OutDataTypeStr=Inherit: Same as input  ParamDataTypeStr=Inherit: Same as input
  Trigonometric Function : Trigonometry  Operator=sincos
  R(v) : Outport  VectorParamsAs1DForOutWhenUnconnected=off
  wires:
  v/1 -> Trigonometric Function/1
  Create 3x3 Matrix/1 -> R(v)/1
  Constant/1 -> Create 3x3 Matrix/8, Create 3x3 Matrix/7, Create 3x3 Matrix/6, Create 3x3 Matrix/3
  Constant1/1 -> Create 3x3 Matrix/9
  Trigonometric Function/2 -> Create 3x3 Matrix/5, Create 3x3 Matrix/1
  Trigonometric Function/1 -> Gain/1, Create 3x3 Matrix/2
  Gain/1 -> Create 3x3 Matrix/4  "-v(1)"

== system MJAUV_Maneuverability_model_V2/MJ-AUV Model & PropulsionSystem/Dynamics and Kinematics/Subsystem9/Subsystem5/{S}->{T} Transformation ==
  v : Inport
  Constant : Constant  Value=0
  Constant1 : Constant
  Create 3x3 Matrix : sharedutil/Create 3x3 Matrix  aMode=aMode
  Gain : Gain  Gain=-1  SaturateOnIntegerOverflow=on  OutDataTypeStr=Inherit: Same as input  ParamDataTypeStr=Inherit: Same as input
  Trigonometric Function : Trigonometry  Operator=sincos
  R(v) : Outport  VectorParamsAs1DForOutWhenUnconnected=off
  wires:
  v/1 -> Trigonometric Function/1
  Create 3x3 Matrix/1 -> R(v)/1
  Constant/1 -> Create 3x3 Matrix/8, Create 3x3 Matrix/7, Create 3x3 Matrix/6, Create 3x3 Matrix/3
  Constant1/1 -> Create 3x3 Matrix/9
  Trigonometric Function/2 -> Create 3x3 Matrix/5, Create 3x3 Matrix/1
  Trigonometric Function/1 -> Gain/1, Create 3x3 Matrix/2
  Gain/1 -> Create 3x3 Matrix/4  "-v(1)"

== system MJAUV_Maneuverability_model_V2/MJ-AUV Model & PropulsionSystem/Dynamics and Kinematics/Subsystem9/Subsystem5/{T}->{F} Transformation ==
  v : Inport
  Constant : Constant  Value=0
  Constant1 : Constant
  Create 3x3 Matrix : sharedutil/Create 3x3 Matrix  aMode=aMode
  Gain : Gain  Gain=-1  SaturateOnIntegerOverflow=on  OutDataTypeStr=Inherit: Same as input  ParamDataTypeStr=Inherit: Same as input
  Trigonometric Function : Trigonometry  Operator=sincos
  R(v) : Outport  VectorParamsAs1DForOutWhenUnconnected=off
  wires:
  Gain/1 -> Create 3x3 Matrix/4  "-v(1)"
  Trigonometric Function/1 -> Create 3x3 Matrix/2, Gain/1
  Trigonometric Function/2 -> Create 3x3 Matrix/1, Create 3x3 Matrix/5
  Constant1/1 -> Create 3x3 Matrix/9
  Constant/1 -> Create 3x3 Matrix/3, Create 3x3 Matrix/6, Create 3x3 Matrix/7, Create 3x3 Matrix/8
  Create 3x3 Matrix/1 -> R(v)/1
  v/1 -> Trigonometric Function/1

== system MJAUV_Maneuverability_model_V2/MJ-AUV Model & PropulsionSystem/Dynamics and Kinematics/Subsystem4/Restoring forces/E1(e)/Skew Symmetrical Operator ==
  v : Inport
  Constant : Constant  Value=0
  Create 3x3 Matrix : sharedutil/Create 3x3 Matrix  aMode=aMode
  Demux : Demux  Outputs=3
      settings: DisplayOption=none
  Gain : Gain  Gain=-1  SaturateOnIntegerOverflow=on  OutDataTypeStr=Inherit: Same as input  ParamDataTypeStr=Inherit: Same as input
  Gain1 : Gain  Gain=-1  SaturateOnIntegerOverflow=on  OutDataTypeStr=Inherit: Same as input  ParamDataTypeStr=Inherit: Same as input
  Gain2 : Gain  Gain=-1  SaturateOnIntegerOverflow=on  OutDataTypeStr=Inherit: Same as input  ParamDataTypeStr=Inherit: Same as input
  S(V) : Outport  VectorParamsAs1DForOutWhenUnconnected=off
  wires:
  Constant/1 -> Create 3x3 Matrix/1, Create 3x3 Matrix/9, Create 3x3 Matrix/5
  Demux/1 -> Gain/1, Create 3x3 Matrix/8  "v(1)"
  Demux/2 -> Gain1/1, Create 3x3 Matrix/3  "v(2)"
  Demux/3 -> Gain2/1, Create 3x3 Matrix/4  "v(3)"
  Gain/1 -> Create 3x3 Matrix/6  "-v(1)"
  Gain1/1 -> Create 3x3 Matrix/7  "-v(2)"
  Gain2/1 -> Create 3x3 Matrix/2  "-v(3)"
  Create 3x3 Matrix/1 -> S(V)/1
  v/1 -> Demux/1

== system MJAUV_Maneuverability_model_V2/MJ-AUV Model & PropulsionSystem/Dynamics and Kinematics/Subsystem4/Rigid-body Coriolis and centripetal matrix/Subsystem/Skew Symmetrical Operator1 ==
  v : Inport
  Constant : Constant  Value=0
  Create 3x3 Matrix : sharedutil/Create 3x3 Matrix  aMode=aMode
  Demux : Demux  Outputs=3
      settings: DisplayOption=none
  Gain : Gain  Gain=-1  SaturateOnIntegerOverflow=on  OutDataTypeStr=Inherit: Same as input  ParamDataTypeStr=Inherit: Same as input
  Gain1 : Gain  Gain=-1  SaturateOnIntegerOverflow=on  OutDataTypeStr=Inherit: Same as input  ParamDataTypeStr=Inherit: Same as input
  Gain2 : Gain  Gain=-1  SaturateOnIntegerOverflow=on  OutDataTypeStr=Inherit: Same as input  ParamDataTypeStr=Inherit: Same as input
  S(V) : Outport  VectorParamsAs1DForOutWhenUnconnected=off
  wires:
  v/1 -> Demux/1
  Create 3x3 Matrix/1 -> S(V)/1
  Gain2/1 -> Create 3x3 Matrix/2  "-v(3)"
  Gain1/1 -> Create 3x3 Matrix/7  "-v(2)"
  Gain/1 -> Create 3x3 Matrix/6  "-v(1)"
  Demux/3 -> Create 3x3 Matrix/4, Gain2/1  "v(3)"
  Demux/2 -> Create 3x3 Matrix/3, Gain1/1  "v(2)"
  Demux/1 -> Create 3x3 Matrix/8, Gain/1  "v(1)"
  Constant/1 -> Create 3x3 Matrix/5, Create 3x3 Matrix/9, Create 3x3 Matrix/1

== system MJAUV_Maneuverability_model_V2/MJ-AUV Model & PropulsionSystem/Dynamics and Kinematics/Subsystem6/Restoring forces1/E1(e)/Skew Symmetrical Operator ==
  v : Inport
  Constant : Constant  Value=0
  Create 3x3 Matrix : sharedutil/Create 3x3 Matrix  aMode=aMode
  Demux : Demux  Outputs=3
      settings: DisplayOption=none
  Gain : Gain  Gain=-1  SaturateOnIntegerOverflow=on  OutDataTypeStr=Inherit: Same as input  ParamDataTypeStr=Inherit: Same as input
  Gain1 : Gain  Gain=-1  SaturateOnIntegerOverflow=on  OutDataTypeStr=Inherit: Same as input  ParamDataTypeStr=Inherit: Same as input
  Gain2 : Gain  Gain=-1  SaturateOnIntegerOverflow=on  OutDataTypeStr=Inherit: Same as input  ParamDataTypeStr=Inherit: Same as input
  S(V) : Outport  VectorParamsAs1DForOutWhenUnconnected=off
  wires:
  v/1 -> Demux/1
  Create 3x3 Matrix/1 -> S(V)/1
  Gain2/1 -> Create 3x3 Matrix/2  "-v(3)"
  Gain1/1 -> Create 3x3 Matrix/7  "-v(2)"
  Gain/1 -> Create 3x3 Matrix/6  "-v(1)"
  Demux/3 -> Create 3x3 Matrix/4, Gain2/1  "v(3)"
  Demux/2 -> Create 3x3 Matrix/3, Gain1/1  "v(2)"
  Demux/1 -> Create 3x3 Matrix/8, Gain/1  "v(1)"
  Constant/1 -> Create 3x3 Matrix/5, Create 3x3 Matrix/9, Create 3x3 Matrix/1

== system MJAUV_Maneuverability_model_V2/MJ-AUV Model & PropulsionSystem/Dynamics and Kinematics/Subsystem6/Rigid-body Coriolis and centripetal matrix1/Subsystem/Skew Symmetrical Operator1 ==
  v : Inport
  Constant : Constant  Value=0
  Create 3x3 Matrix : sharedutil/Create 3x3 Matrix  aMode=aMode
  Demux : Demux  Outputs=3
      settings: DisplayOption=none
  Gain : Gain  Gain=-1  SaturateOnIntegerOverflow=on  OutDataTypeStr=Inherit: Same as input  ParamDataTypeStr=Inherit: Same as input
  Gain1 : Gain  Gain=-1  SaturateOnIntegerOverflow=on  OutDataTypeStr=Inherit: Same as input  ParamDataTypeStr=Inherit: Same as input
  Gain2 : Gain  Gain=-1  SaturateOnIntegerOverflow=on  OutDataTypeStr=Inherit: Same as input  ParamDataTypeStr=Inherit: Same as input
  S(V) : Outport  VectorParamsAs1DForOutWhenUnconnected=off
  wires:
  v/1 -> Demux/1
  Create 3x3 Matrix/1 -> S(V)/1
  Gain2/1 -> Create 3x3 Matrix/2  "-v(3)"
  Gain1/1 -> Create 3x3 Matrix/7  "-v(2)"
  Gain/1 -> Create 3x3 Matrix/6  "-v(1)"
  Demux/3 -> Create 3x3 Matrix/4, Gain2/1  "v(3)"
  Demux/2 -> Create 3x3 Matrix/3, Gain1/1  "v(2)"
  Demux/1 -> Create 3x3 Matrix/8, Gain/1  "v(1)"
  Constant/1 -> Create 3x3 Matrix/5, Create 3x3 Matrix/9, Create 3x3 Matrix/1

== system MJAUV_Maneuverability_model_V2/MJ-AUV Model & PropulsionSystem/Dynamics and Kinematics/Subsystem6/Subsystem1/Quaternion normalisation/norm 1x4 vector ==
  Inport : Inport
  Plus : Sum  Inputs=++++
  Selector : Selector  InputPortWidth=4  IndexOptions=Index vector (dialog)  Indices=[1]  OutputSizes=1
  Selector1 : Selector  InputPortWidth=4  IndexOptions=Index vector (dialog)  Indices=[2]  OutputSizes=1
  Selector2 : Selector  InputPortWidth=4  IndexOptions=Index vector (dialog)  Indices=[3]  OutputSizes=1
  Selector3 : Selector  InputPortWidth=4  IndexOptions=Index vector (dialog)  Indices=[4]  OutputSizes=1
  Sqrt : Sqrt
  Square{,1..3} (4 alike) : Math  Operator=square  SignedPower=on
  norm : Outport  VectorParamsAs1DForOutWhenUnconnected=off
  wires:
  Selector/1 -> Square/1
  Selector1/1 -> Square1/1
  Sqrt/1 -> norm/1
  Selector2/1 -> Square2/1
  Plus/1 -> Sqrt/1
  Selector3/1 -> Square3/1
  Square3/1 -> Plus/4
  Inport/1 -> Selector1/1, Selector/1, Selector2/1, Selector3/1
  Square/1 -> Plus/1
  Square1/1 -> Plus/2
  Square2/1 -> Plus/3

== system MJAUV_Maneuverability_model_V2/MJ-AUV Model & PropulsionSystem/Dynamics and Kinematics/Subsystem7/Restoring forces1/E1(e)/Skew Symmetrical Operator ==
  v : Inport
  Constant : Constant  Value=0
  Create 3x3 Matrix : sharedutil/Create 3x3 Matrix  aMode=aMode
  Demux : Demux  Outputs=3
      settings: DisplayOption=none
  Gain : Gain  Gain=-1  SaturateOnIntegerOverflow=on  OutDataTypeStr=Inherit: Same as input  ParamDataTypeStr=Inherit: Same as input
  Gain1 : Gain  Gain=-1  SaturateOnIntegerOverflow=on  OutDataTypeStr=Inherit: Same as input  ParamDataTypeStr=Inherit: Same as input
  Gain2 : Gain  Gain=-1  SaturateOnIntegerOverflow=on  OutDataTypeStr=Inherit: Same as input  ParamDataTypeStr=Inherit: Same as input
  S(V) : Outport  VectorParamsAs1DForOutWhenUnconnected=off
  wires:
  Constant/1 -> Create 3x3 Matrix/1, Create 3x3 Matrix/9, Create 3x3 Matrix/5
  Demux/1 -> Gain/1, Create 3x3 Matrix/8  "v(1)"
  Demux/2 -> Gain1/1, Create 3x3 Matrix/3  "v(2)"
  Demux/3 -> Gain2/1, Create 3x3 Matrix/4  "v(3)"
  Gain/1 -> Create 3x3 Matrix/6  "-v(1)"
  Gain1/1 -> Create 3x3 Matrix/7  "-v(2)"
  Gain2/1 -> Create 3x3 Matrix/2  "-v(3)"
  Create 3x3 Matrix/1 -> S(V)/1
  v/1 -> Demux/1

== system MJAUV_Maneuverability_model_V2/MJ-AUV Model & PropulsionSystem/Dynamics and Kinematics/Subsystem7/Rigid-body Coriolis and centripetal matrix1/Subsystem/Skew Symmetrical Operator1 ==
  v : Inport
  Constant : Constant  Value=0
  Create 3x3 Matrix : sharedutil/Create 3x3 Matrix  aMode=aMode
  Demux : Demux  Outputs=3
      settings: DisplayOption=none
  Gain : Gain  Gain=-1  SaturateOnIntegerOverflow=on  OutDataTypeStr=Inherit: Same as input  ParamDataTypeStr=Inherit: Same as input
  Gain1 : Gain  Gain=-1  SaturateOnIntegerOverflow=on  OutDataTypeStr=Inherit: Same as input  ParamDataTypeStr=Inherit: Same as input
  Gain2 : Gain  Gain=-1  SaturateOnIntegerOverflow=on  OutDataTypeStr=Inherit: Same as input  ParamDataTypeStr=Inherit: Same as input
  S(V) : Outport  VectorParamsAs1DForOutWhenUnconnected=off
  wires:
  v/1 -> Demux/1
  Create 3x3 Matrix/1 -> S(V)/1
  Gain2/1 -> Create 3x3 Matrix/2  "-v(3)"
  Gain1/1 -> Create 3x3 Matrix/7  "-v(2)"
  Gain/1 -> Create 3x3 Matrix/6  "-v(1)"
  Demux/3 -> Create 3x3 Matrix/4, Gain2/1  "v(3)"
  Demux/2 -> Create 3x3 Matrix/3, Gain1/1  "v(2)"
  Demux/1 -> Create 3x3 Matrix/8, Gain/1  "v(1)"
  Constant/1 -> Create 3x3 Matrix/5, Create 3x3 Matrix/9, Create 3x3 Matrix/1
